simulink model "smmodel"  (R2021a)
settings: Solver=ode23tb  StartTime=0.0  StopTime=5  FixedStep=0.00001  RelTol=1e-3
PreLoadFcn:
  | x-d=1;
values from neighbouring files (symbols this model uses):
  Cf = 1e-4    (= 0.0001)    [Data.m]
  Ibase = Ibase*sqrt(2)    [Data.m]
  Lc = 0.00125    [Data.m]
  Lf = 0.1    [Data.m]
  Rc = 0.01    [Data.m]
  Rf = 0.01    [Data.m]
  Vbase = Vbase*sqrt(2)    [Data.m]
  Vdc = sqrt(2)*100    [Data.m]
libraries: spsIGBTDiodeLib x6, spsThreePhaseSeriesRLCBranchLib x3, simulink x2, spsabctodq0Lib x2, spsDCVoltageSourceLib x1, spsThreePhaseVIMeasurementLib x1, spsGroundLib x1, spsThreePhaseSeriesRLCLoadLib x1, spsdq0toabcLib x1, spspowerguiLib x1
settings Model: Creator=udipb  LastModifiedBy=Electrical
settings SolverCC: AlgebraicLoopSolver=TrustRegion
settings DataIOCC: ReturnWorkspaceOutputs=off
settings DebuggingCC: SFMachineParentedDataDiag=warning  ArithmeticOperatorsInVariantConditions=warning
settings SFSimCC: SimUseLocalCustomCode=off  CustomCodeUndefinedFunction=UseInterfaceOnly
settings RTWCC: RTWUseLocalCustomCode=off

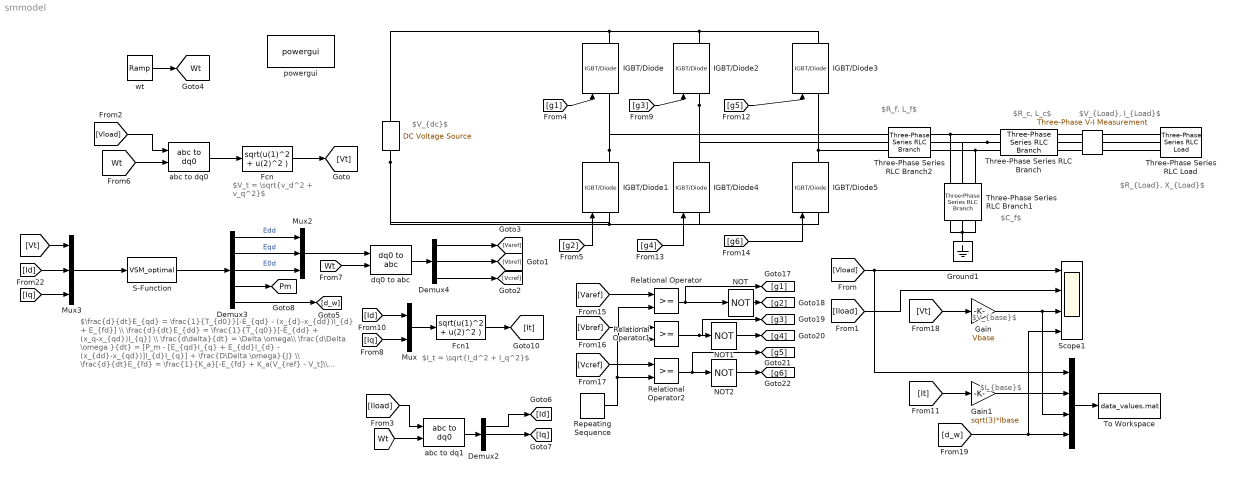
== system smmodel ==
  note: $R_f, L_f$
  note: $\frac{d}{dt}E_{qd} = \frac{1}{T_{d0}}[-E_{qd} - (x_{d}-x_{dd})I_{d} + E_{fd}] \\ \frac{d}{dt}E_{dd} = \frac{1}{T_{q0}}[-E_{dd} + (x_q-x_{qd})I_{q}] \\ \frac{d\delta}{dt} = \Delta \omega\\ \frac{d\Delta \omega }{dt} = [P_m - [E_{qd}I_{q} + E_{dd}I_{d} - (x_{dd}-x_{qd})]I_{d}I_{q}] + \frac{D\Delta \omega}{J} \\ \frac{d}{dt}E_{fd} = \frac{1}{K_a}[-E_{fd} + K_a(V_{ref} - V_t]\\ \frac{d}{dt}P_{sv} = \frac{1}{T_{sv}}[-P_{sv} + P_{ref} - \Delta \omega/R_d] \\ \frac{d}{dt}P_m = \frac{1}{T_{ch}}[-P_m + P_{sv}]$
  note: $V_t = \sqrt{v_d^2 + v_q^2}$
  note: $C_f$
  note: $R_c, L_c$
  note: $R_{Load}, X_{Load}$
  note: $V_{Load}, I_{Load}$
  note: $V_{dc}$
  note: $I_t = \sqrt{I_d^2 + I_q^2}$
  note: $V_{base}$
  note: $I_{base}$
  "      " : Mux
  "                   " : spsDCVoltageSourceLib/DC Voltage Source  Amplitude=Vdc  Measurements=None
  "                           " : spsThreePhaseVIMeasurementLib/Three-Phase V-I Measurement  VoltageMeasurement=phase-to-phase  SetLabelV=on  LabelV=Vload  Vpu=on  VpuLL=off  CurrentMeasurement=yes  SetLabelI=on  LabelI=Iload  Ipu=on  Pbase=1e3  Vbase=400  OutputType=Complex  PhasorSimulation=off  PSBequivalent=0
  Demux2 : Demux  Outputs=3
  Demux3 : Demux  Outputs=5
  Demux4 : Demux  Outputs=3
  Fcn : Fcn  Expr=sqrt(u(1)^2 + u(2)^2 )
  Fcn1 : Fcn  Expr=sqrt(u(1)^2 + u(2)^2 )
  Gain : Gain  Gain=Vbase
  Gain1 : Gain  Gain=sqrt(3)*Ibase
  Ground1 : spsGroundLib/Ground  LConnTagsString=a
  IGBT/Diode{,1..5} (6 alike) : spsIGBTDiodeLib/IGBT//Diode  Ron=1e-3  Rs=1e5  Cs=inf  Measurements=on
  Mux : Mux  Inputs=2
  Mux2 : Mux  Inputs=3
  Mux3 : Mux  Inputs=3
  NOT : Logic  Operator=NOT  IconShape=distinctive  AllPortsSameDT=off  OutDataTypeStr=boolean
  NOT1 : Logic  Operator=NOT  IconShape=distinctive  AllPortsSameDT=off  OutDataTypeStr=boolean
  NOT2 : Logic  Operator=NOT  IconShape=distinctive  AllPortsSameDT=off  OutDataTypeStr=boolean
  Relational Operator : RelationalOperator  OutDataTypeStr=boolean  RndMeth=Simplest
  Relational Operator1 : RelationalOperator  OutDataTypeStr=boolean  RndMeth=Simplest
  Relational Operator2 : RelationalOperator  OutDataTypeStr=boolean  RndMeth=Simplest
  Repeating Sequence : simulink/Sources/Repeating Sequence  rep_seq_t=[0 0.00005 0.0001]  rep_seq_y=[-1 1 -1]
  S-Function : S-Function  FunctionName=VSM_optimal  SFunctionDeploymentMode=off  EnableBusSupport=off
  Scope1 : Scope  NumInputPorts=4
  Three-Phase Series RLC Branch : spsThreePhaseSeriesRLCBranchLib/Three-Phase Series RLC Branch  LConnTagsString=A|B|C  RConnTagsString=A|B|C  BranchType=RL  Resistance=Rc  Inductance=Lc  Capacitance=1e-6  Measurements=None
  Three-Phase Series RLC Branch1 : spsThreePhaseSeriesRLCBranchLib/Three-Phase Series RLC Branch  LConnTagsString=A|B|C  RConnTagsString=A|B|C  BranchType=C  Resistance=Rc  Inductance=Lc  Capacitance=Cf  Measurements=None
  Three-Phase Series RLC Branch2 : spsThreePhaseSeriesRLCBranchLib/Three-Phase Series RLC Branch  LConnTagsString=A|B|C  RConnTagsString=A|B|C  BranchType=RL  Resistance=Rf  Inductance=Lf  Capacitance=1e-6  Measurements=None
  Three-Phase Series RLC Load : spsThreePhaseSeriesRLCLoadLib/Three-Phase Series RLC Load  LConnTagsString=A|B|C  Configuration=Y (grounded)  NominalVoltage=400  Vabc=[1e3 1e3 1e3]  Vabcp=[1e3 1e3 1e3]  NominalFrequency=50  UnbalancedPower=off  ActivePower=800  InductivePower=600  CapacitivePower=0  Pabc=[10e3 9e3 11e3]  QLabc=[100 90 110]  QCabc=[100 90 110]  Pabcp=[10e3 9e3 11e3]  QLabcp=[100 90 110]  QCabcp=[100 90 110]  Measurements=None  LoadType=constant Z
  To Workspace : ToFile  Filename=data_values.mat  MatrixName=Data
  abc to dq0 : spsabctodq0Lib/abc to dq0  Alignment=Aligned with phase A axis
  abc to dq1 : spsabctodq0Lib/abc to dq0  Alignment=Aligned with phase A axis
  dq0 to abc : spsdq0toabcLib/dq0 to abc  Alignment=Aligned with phase A axis
  powergui : spspowerguiLib/powergui  Priority=1  SimulationMode=Discrete  SampleTime=0.00001  frequency=60  Iterations=50  frequencyindice=0  Pbase=100e6  ErrMax=1e-4  UnitsV=kV  UnitsW=MW  buscounter=0  FunctionMessages=off  echomessages=off  EnableUseOfTLC=off  CurrentSourceSwitches=off  DisableSnubberDevices=on  DisableRonSwitches=on  DisableVfSwitches=on  DisplayEquations=off  AutomaticDiscreteSolvers=off  SolverType=Tustin/Backward Euler (TBE)  Interpol=off  ExternalGateDelay=off  methode=off  Ts=100  x0status=zero  SPID=on  SwTol=0  HookPort=off  NonlinearTolerance=1e-4  nMaxIteration=100  ContinueOnMaxIteration=off  RestoreLinks=warning  ResistiveCurrentMeasurement=off  Frange=[0:2:500]  Ylog=off  Xlog=on  ShowGrid=off  save=off  variable=ZData  structure=0  ZoomFFT=off  StartTime=0.0  cycles=1  DisplayStyle=1  fundamental=60  FreqAxis=off  MaxFrequency=1000  frequencyindicesteady=1  RmsSteady=1  display=off
  wt : simulink/Sources/Ramp  slope=2*pi*50  start=0  InitialOutput=0
  tag scope: Pm=global, Wt=global
  wires:
  Fcn/1 -> [Vt]
  abc to dq0/1 -> Fcn/1
  [Wt] -> abc to dq0/2
  [Wt] -> abc to dq1/2
  abc to dq1/1 -> Demux2/1
  Demux2/1 -> [Id]
  Demux2/2 -> [Iq]
  [Vload] -> abc to dq0/1
  [Iload] -> abc to dq1/1
  [g1] -> IGBT/Diode/1
  [g2] -> IGBT/Diode1/1
  [g3] -> IGBT/Diode2/1
  [g4] -> IGBT/Diode4/1
  [g5] -> IGBT/Diode3/1
  [g6] -> IGBT/Diode5/1
  [Vt] -> Gain/1
  [d_w] -> Scope1/4, "      "/4
  wt/1 -> [Wt]
  [Iload] -> Scope1/2
  [Vload] -> "      "/1, Scope1/1
  Demux4/1 -> [Varef]
  Demux4/2 -> [Vbref]
  Demux4/3 -> [Vcref]
  "      "/1 -> To Workspace/1
  Relational Operator1/1 -> [g3], NOT1/1
  [Varef] -> Relational Operator/1
  [Vcref] -> Relational Operator2/1
  NOT2/1 -> [g6]
  [Vbref] -> Relational Operator1/1
  NOT1/1 -> [g4]
  Relational Operator/1 -> [g1], NOT/1
  NOT/1 -> [g2]
  Repeating Sequence/1 -> Relational Operator/2, Relational Operator1/2, Relational Operator2/2
  Relational Operator2/1 -> [g5], NOT2/1
  Demux3/5 -> [d_w]
  Demux3/4 -> [Pm]
  Mux3/1 -> S-Function/1
  [Id] -> Mux3/2
  [Iq] -> Mux3/3
  Mux2/1 -> dq0 to abc/1
  S-Function/1 -> Demux3/1
  dq0 to abc/1 -> Demux4/1
  Demux3/1 -> Mux2/1  "Edd"
  [Vt] -> Mux3/1
  Demux3/3 -> Mux2/3  "E0d"
  Demux3/2 -> Mux2/2  "Eqd"
  [Wt] -> dq0 to abc/2
  Gain/1 -> "      "/3, Scope1/3
  Mux/1 -> Fcn1/1
  [Id] -> Mux/1
  [Iq] -> Mux/2
  Fcn1/1 -> [It]
  [It] -> Gain1/1
  Gain1/1 -> "      "/2
  connections:
  "                   "/RConn1 -- IGBT/Diode1/LConn1 -- IGBT/Diode5/LConn1 -- IGBT/Diode4/LConn1
  IGBT/Diode1/RConn1 -- IGBT/Diode/LConn1 -- Three-Phase Series RLC Branch2/LConn1
  IGBT/Diode3/LConn1 -- Three-Phase Series RLC Branch2/LConn3 -- IGBT/Diode5/RConn1
  IGBT/Diode2/RConn1 -- IGBT/Diode/RConn1 -- "                   "/LConn1 -- IGBT/Diode3/RConn1
  IGBT/Diode2/LConn1 -- Three-Phase Series RLC Branch2/LConn2 -- IGBT/Diode4/RConn1
  Three-Phase Series RLC Branch/LConn3 -- Three-Phase Series RLC Branch1/LConn3 -- Three-Phase Series RLC Branch2/RConn3
  Three-Phase Series RLC Branch/RConn1 -- "                           "/LConn1
  Three-Phase Series RLC Branch/LConn1 -- Three-Phase Series RLC Branch1/LConn1 -- Three-Phase Series RLC Branch2/RConn1
  "                           "/LConn2 -- Three-Phase Series RLC Branch/RConn2
  Three-Phase Series RLC Branch/RConn3 -- "                           "/LConn3
  Three-Phase Series RLC Branch/LConn2 -- Three-Phase Series RLC Branch2/RConn2 -- Three-Phase Series RLC Branch1/LConn2
  Three-Phase Series RLC Branch1/RConn1 -- Three-Phase Series RLC Branch1/RConn3 -- Ground1/LConn1 -- Three-Phase Series RLC Branch1/RConn2
  Three-Phase Series RLC Load/LConn1 -- "                           "/RConn1
  Three-Phase Series RLC Load/LConn2 -- "                           "/RConn2
  Three-Phase Series RLC Load/LConn3 -- "                           "/RConn3
